simulink model "LED_Cmd_varZ_eqHarness_req"  (Simulink 7.9)
settings: Solver=FixedStepDiscrete  StartTime=0.0  StopTime=10  RelTol=1e-3
PreLoadFcn:
  | LED_Cmd_varZ_selfinit
undefined symbols (not defined in the file): sigbuilder_block
libraries: simulink x1
CloseFcn:
  | rtwprivate ssgencode ModelCloseRequest ADL
settings Model: RequirementInfo="{}  %GIDa_ffb28f1c_3982_4734_9f04_bbd4c8d0ce22"  MinMaxOverflowLogging=ForceOff  SldvGeneratedHarnessModel=TestUnitModel=LED_Cmd_varZ|  Creator=fguerin  LastModifiedBy=klindqvi  CovMetricSettings=dcmoe  CovHTMLOptions=-aTS=1 -bRG=1 -bTC=0 -hTR=0 -nFC=0 -scm=1 -bcm=1  covSaveCumulativeToWorkspaceVar=off  CovSaveSingleToWorkspaceVar=off  CovModelRefEnable=on  CovExternalEMLEnable=on
settings DataIOCC: ExternalInput=SIM_LockDoorRequest  LimitDataPoints=off  SaveFormat=StructureWithTime  SaveOutput=off  DSMLogging=off  SaveTime=off  SignalLoggingName=logsOut
settings OptimizationCC: InlineParams=on  InlineInvariantSignals=on  EnhancedBackFolding=on  ZeroExternalMemoryAtStartup=off  ZeroInternalMemoryAtStartup=off  EfficientFloat2IntCast=on  OptimizeModelRefInitCode=on  LifeSpan=1
settings DebuggingCC: ReadBeforeWriteMsg=EnableAllAsError  WriteAfterWriteMsg=EnableAllAsError  WriteAfterReadMsg=EnableAllAsError  AlgebraicLoopMsg=error  ArtificialAlgebraicLoopMsg=error  SaveWithDisabledLinksMsg=error  SaveWithParameterizedLinksMsg=error  CheckSSInitialOutputMsg=off  CheckExecutionContextPreStartOutputMsg=on  CheckExecutionContextRuntimeOutputMsg=on  BlockPriorityViolationMsg=error  SolverPrmCheckMsg=none  InheritedTsInSrcMsg=none  MultiTaskCondExecSysMsg=warning  MultiTaskRateTransMsg=warning  IntegerOverflowMsg=none  ParameterUnderflowMsg=error  ParameterPrecisionLossMsg=error  ParameterTunabilityLossMsg=error  UnnecessaryDatatypeConvMsg=warning  VectorMatrixConversionMsg=error  SignalLabelMismatchMsg=warning  SFcnCompatibilityMsg=error  BusObjectLabelMismatch=error  RootOutportRequireBusObject=error  AssertControl=DisableAll  ModelReferenceIOMsg=error  ModelReferenceIOMismatchMessage=error  ModelReferenceCSMismatchMessage=warning  UnknownTsInhSupMsg=error  ModelReferenceDataLoggingMessage=error  ModelReferenceSymbolNameMessage=none  StrictBusMsg=ErrorOnBusTreatedAsVector
settings HardwareCC: ProdLargestAtomicInteger=Long  ProdLargestAtomicFloat=Double  ProdIntDivRoundTo=Zero  ProdEndianess=BigEndian  ProdHWDeviceType=Freescale->MPC5500
settings ModelReferenceCC: ModelReferenceNumInstancesAllowed=Single
settings SFSimCC: SimParseCustomCode=off
settings RTWCC: SystemTargetFile=ert.tlc  TemplateMakefile=ert_default_tmf  Description=Embedded Coder  GenerateReport=on  RTWVerbose=off  ProcessScript=ert_make_rtw_hook  IncludeHyperlinkInReport=on  GenerateTraceInfo=on  GenerateTraceReport=on  GenerateTraceReportSl=on  GenerateTraceReportSf=on  GenerateTraceReportEml=on  GenerateCodeMetricsReport=on
settings MATStruct: className=rtw.pil.Bullseye  argsAllComponents=[]  excludedModels=[]  includeReferencedModels=on  includeTopModel=on  enabled=off
settings CodeAppCC: ForceParamTrailComments=on  IgnoreCustomStorageClasses=off  IgnoreTestpoints=on  MangleLength=4  InlinedPrmAccess=Macros  ReqsInCode=on
settings ERTTargetCC: CodeReplacementLibrary=ANSI_C  MultiwordLength=2048  SupportAbsoluteTime=off  SupportNonFinite=off  SupportComplex=off  PortableWordSizes=on  InlinedParameterPlacement=NonHierarchical  ERTCustomFileTemplate=example_file_process.tlc  ConvertIfToSwitch=off  SuppressUnreachableDefaultCases=off
settings ConfigComp: Description=Design Verifier Custom Configuration Component  DVMaxProcessTime=600  DVDisplayUnsatisfiableObjectives=on  DVAutomaticStubbing=off  DVOutputDir=C:\work\Presentations\ISO26262_workshop\newsandbox\iso26262package\WorkProducts\CodeTest  DVMakeOutputFilesUnique=off  DVModelCoverageObjectives=MCDC  DVTestSuiteOptimization=CombinedObjectives  DVDataFileName=LED_Cmd_varZ_sldvdata.mat  DVHarnessModelFileName=C:\work\Presentations\ISO26262_workshop\newsandbox\iso26262package\WorkProducts\CodeTest\LED_Cmd_varZ_eqHarness  DVModelReferenceHarness=on  DVSaveReport=on  DVReportFileName=LED_Cmd_varZ_SLDV.html  DVDisplayReport=off

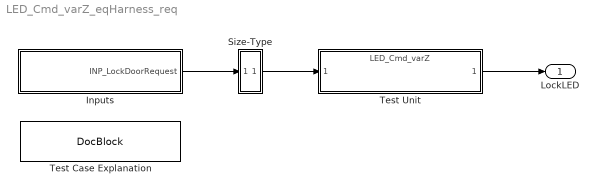
== system LED_Cmd_varZ_eqHarness_req ==
  Inputs : Subsystem  Tag=STV Subsys  LoadFcn=sigbuilder_block('load');  StartFcn=sigbuilder_block('start');  StopFcn=sigbuilder_block('stop');  ClipboardFcn=sigbuilder_block('clipboard');  mask(Sigbuilder block){}
      mask init:
      | if ~strcmp(get_param(bdroot(gcb),'SimulationStatus'),'stopped'),tuvar = sigbuilder_block('maskInit'); end
      settings: CopyFcn=sigbuilder_block('copy');  DeleteFcn=sigbuilder_block('delete');  ModelCloseFcn=sigbuilder_block('modelClose');  PreSaveFcn=sigbuilder_block('preSave');  PauseFcn=sigbuilder_block('pause')  ContinueFcn=sigbuilder_block('continue')  NameChangeFcn=sigbuilder_block('namechange');  OpenFcn=sigbuilder_block('open',[88.5 153.75 519.75 399.75 ]);  CloseFcn=sigbuilder_block('close');
      mask Display: plot(0, 0, 100, 100,[2, 2, 32, 32, 2], [68, 8, 8, 68, 68],[32, 2], [38, 38], [32, 19, 2],[53, 60, 44], [32, 17, 17, 2],[16, 16, 31, 31]);txt = getActiveGroup(gcbh);text(2, 100, txt,'verticalAlignment', 'top');
  Size-Type : Subsystem
  Test Case Explanation : simulink/Model-Wide Utilities/DocBlock  DocumentType=Text
  Test Unit : ModelReference  ModelNameDialog=LED_Cmd_varZ  SimulationMode=Normal  ModelReferenceVersion=1.365  CopyOfModelName=LED_Cmd_varZ  DefaultDataLogging=off
  LockLED : Outport  OutDataTypeStr=boolean  PortDimensions=1
  wires:
  Inputs/1(INP_LockDoorRequest) -> Size-Type/1(In1)
  Size-Type/1(Out1) -> Test Unit/1
  Test Unit/1 -> LockLED/1

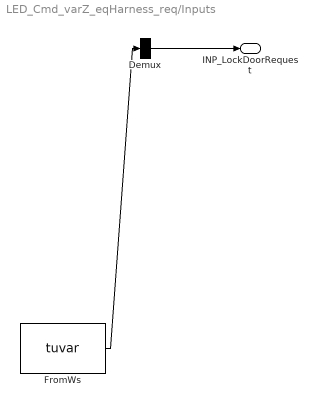
== system LED_Cmd_varZ_eqHarness_req/Inputs ==
  Demux : Demux  Tag=STV Demux  Outputs=1
  FromWs : FromWorkspace  Tag=STV FromWs  VariableName=tuvar  SampleTime=0  SigBuilderData=DataTag0  VnvData=DataTag1
      SigBuilderData=|
      | dataSet(1).timeRange = [0 10]
      | dataSet(1).name = 'Test1'
      | dataSet(2).timeRange = [0 10]
      | dataSet(2).name = 'Test2'
      | dataSet(3).timeRange = [0 10]
      | dataSet(3).name = 'Test3'
      | sbobj.Name = 'Signal Builder'
      | sbobj.Groups(1).Name = 'Test1'
      | sbobj.Groups(1).Signals.Name = 'INP_LockDoorRequest'
      | sbobj.Groups(1).Signals.XData = [0 10]
      | sbobj.Groups(1).Signals.YData = [0 0]
      | sbobj.Groups(2).Name = 'Test2'
      | sbobj.Groups(2).Signals.Name = 'INP_LockDoorRequest'
      | sbobj.Groups(2).Signals.XData = [0 1 2 3 4 5 6 7 8 9 10]
      | sbobj.Groups(2).Signals.YData = [0 1 1 1 1 1 1 1 1 1 1]
      | sbobj.Groups(3).Name = 'Test3'
      | sbobj.Groups(3).Signals.Name = 'INP_LockDoorRequest'
      | sbobj.Groups(3).Signals.XData = [0 1 2 10]
      | sbobj.Groups(3).Signals.YData = [0 1 0 0]
  INP_LockDoorRequest : Outport
  wires:
  FromWs/1 -> Demux/1
  Demux/1 -> INP_LockDoorRequest/1

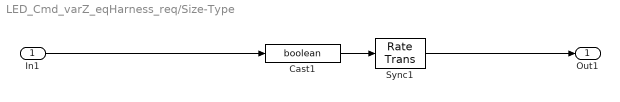
== system LED_Cmd_varZ_eqHarness_req/Size-Type ==
  In1 : Inport
  Cast1 : DataTypeConversion  OutDataTypeStr=boolean  SaturateOnIntegerOverflow=on  RndMeth=Zero
  Sync1 : RateTransition  OutPortSampleTime=[0.20000000000000001,0]
  Out1 : Outport
  wires:
  In1/1 -> Cast1/1
  Cast1/1 -> Sync1/1
  Sync1/1 -> Out1/1
